simulink model "InterferenceModelingExample"  (Simulink 10.1)
settings: Solver=FixedStepDiscrete  StartTime=0.0  StopTime=1  RelTol=1e-3
undefined symbols (not defined in the file or in its folder): designMultirateFIR
libraries: commrflib2 x8, commdigbbndpm3 x2, commfilt2 x2, commrandsrc3 x2, commsink2 x1, commrfcorlib x1, commsync2 x1, commdigbbndcpm2 x1, dspsigattribs x1, dspmlti4 x1
settings Model: Creator=The MathWorks, Inc.  LastModifiedBy=iba
settings DataIOCC: SaveFormat=Dataset  ReturnWorkspaceOutputs=on
settings OptimizationCC: EfficientMapNaN2IntZero=off  LifeSpan=auto
settings DebuggingCC: UnderspecifiedInitializationDetection=Simplified  MergeDetectMultiDrivingBlocksExec=error  SFUnexpectedBacktrackingDiag=error  SFNoUnconditionalDefaultTransitionDiag=error  SFExecutionAtInitializationDiag=warning  ArithmeticOperatorsInVariantConditions=error
settings HardwareCC: ProdBitPerPointer=64  ProdBitPerSizeT=64  ProdBitPerPtrDiffT=64  ProdLargestAtomicFloat=Float  ProdIntDivRoundTo=Zero  ProdEndianess=LittleEndian  ProdWordSize=64  ProdHWDeviceType=Intel->x86-64 (Windows64)  TargetBitPerPointer=64  TargetBitPerSizeT=64  TargetBitPerPtrDiffT=64  TargetLongLongMode=on  TargetIntDivRoundTo=Zero  TargetEndianess=LittleEndian  TargetWordSize=64  TargetHWDeviceType=MATLAB Host  ProdEqTarget=off
settings ModelReferenceCC: PropagateSignalLabelsOutOfModel=on
settings SFSimCC: SimUseLocalCustomCode=on
settings RTWCC: RTWUseLocalCustomCode=on
settings CodeAppCC: MaxIdLength=128  StateflowObjectComments=off
settings ConfigComp: CovMetricSettings=dwe  CovHtmlReporting=off  CovSaveCumulativeToWorkspaceVar=off  CovSaveSingleToWorkspaceVar=off  CovExternalEMLEnable=on

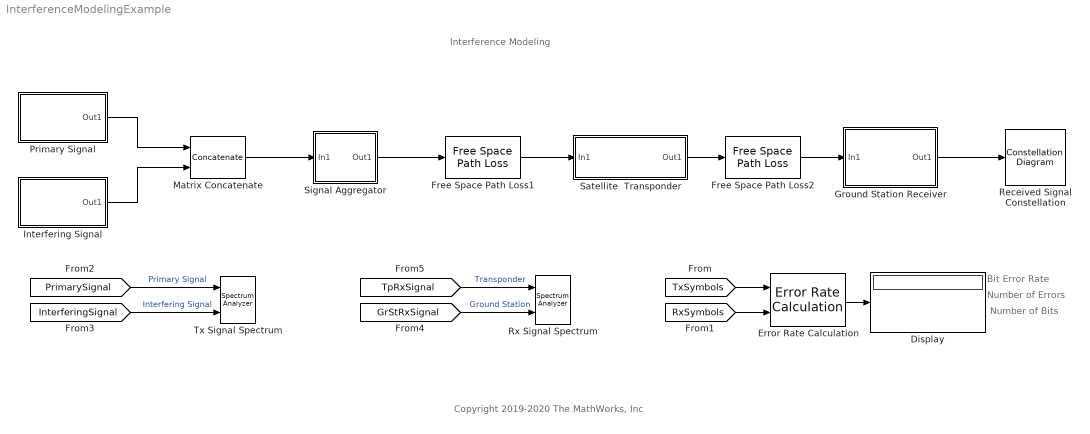
== system InterferenceModelingExample ==
  note: Interference Modeling
  note: Copyright 2019-2020 The MathWorks, Inc
  note: Bit Error Rate
  note: Number of Errors
  note: Number of Bits
  Display : Display
  Error Rate Calculation : commsink2/Error Rate Calculation  N=16 % 10  st_delay=0  cp_mode=Entire frame  subframe=[]  PMode=Port  WsName=ErrorVec  RsMode2=off  stop=off  numErr=100  maxBits=1e6
  Free Space Path Loss1 : commrflib2/Free Space Path Loss  mode=Decibels  dB=200  d=0.100  fc=1920
      settings: SourceProductBaseCode=CM
  Free Space Path Loss2 : commrflib2/Free Space Path Loss  mode=Decibels  dB=200  d=0.100  fc=1920
      settings: SourceProductBaseCode=CM
  Ground Station Receiver : Subsystem
      mask Display: disp('Ground Station\nReceiver')
  Interfering Signal : Subsystem
      mask Display: disp('Interfering\nSignal')
  Matrix Concatenate : Concatenate  Mode=Multidimensional array  ConcatenateDimension=2
  Primary Signal : Subsystem
      mask Display: disp('Primary\nSignal')
  Received Signal Constellation : ConstellationDiagram
  Rx Signal Spectrum : SpectrumAnalyzer  NumInputPorts=2
  Satellite  Transponder : Subsystem
      mask Display: disp('Satellite\nTransponder')
  Signal Aggregator : Subsystem  mask(Signal Aggregator){InterpolationMode=Auto, InputSampleRate=1e6, CenterFrequency=[0 400e3]}
      mask prompts: InterpolationMode "Interpolation mode:"; InputSampleRate "Sample rate of input signal (Hz):"; CenterFrequency "Desired output center frequencys (Hz):"
      mask help: Frequency shift input signals and aggregate them. Optionally, before frequency shifting the input signals, interpolate them such that the bandwidth of the aggregate output signal includes all the input signals.
      mask init:
      | Lnew = signalAggregator_MaskInit(gcbh, 'init', InterpolationMode, ...
      |     InputSampleRate, CenterFrequency);
      mask TypeOptions InterpolationMode: None | Auto
      mask Callback InterpolationMode: signalAggregator_MaskInit(gcbh, 'interpolationMode');
      mask Display: disp('Signal\nAggregator')
  Tx Signal Spectrum : SpectrumAnalyzer  NumInputPorts=2
  wires:
  Error Rate Calculation/1 -> Display/1
  Signal Aggregator/1(Out1) -> Free Space Path Loss1/1
  Free Space Path Loss1/1 -> Satellite  Transponder/1(In1)
  Satellite  Transponder/1(Out1) -> Free Space Path Loss2/1
  Ground Station Receiver/1(Out1) -> Received Signal Constellation/1
  [PrimarySignal] -> Tx Signal Spectrum/1  "Primary Signal"
  [InterferingSignal] -> Tx Signal Spectrum/2  "Interfering Signal"
  Primary Signal/1(Out1) -> Matrix Concatenate/1
  Interfering Signal/1(Out1) -> Matrix Concatenate/2
  Matrix Concatenate/1 -> Signal Aggregator/1(In1)
  [RxSymbols] -> Error Rate Calculation/2
  [TxSymbols] -> Error Rate Calculation/1
  [TpRxSignal] -> Rx Signal Spectrum/1  "Transponder"
  Free Space Path Loss2/1 -> Ground Station Receiver/1(In1)
  [GrStRxSignal] -> Rx Signal Spectrum/2  "Ground Station"

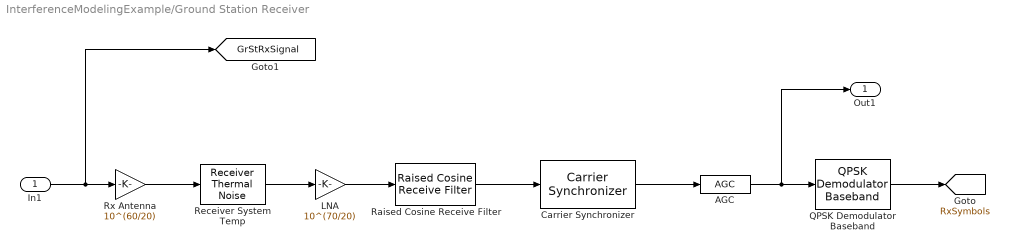
== system InterferenceModelingExample/Ground Station Receiver ==
  In1 : Inport
  AGC : commrfcorlib/AGC  LegacyMode=off  DetectorMethod=Rectifier  LoopMethod=Linear  UpdatePeriod=100  StepSize=0.1  AdaptationStepSize=0.01  DesiredOutputPower=1  AveragingLength=200  MaximumGain=30  MaxPowerGain=60  GainOutputPort=off  InputPowerOutputPort=off  SimulateUsing=Interpreted execution
  Carrier Synchronizer : commsync2/Carrier Synchronizer  Modulation=QPSK  ModulationPhaseOffset=Auto  CustomPhaseOffset=0  SamplesPerSymbol=1  DampingFactor=0.707  NormalizedLoopBandwidth=0.01  EstimatedPhaseErrorOutputPort=off  SimulateUsing=Code generation
  LNA : Gain  Gain=10^(70/20)
  QPSK Demodulator Baseband : commdigbbndpm3/QPSK Demodulator Baseband  OutType=Integer  DecType=Log-likelihood ratio  VarSource=Dialog  Variance=1  Dec=Gray  Ph=pi/4  outDtype1=Inherit via internal rule  outDtype2=Inherit via internal rule  derotateFactorWordLen=16  derotateFactorDataTypeStr=Inherit: Same word length as input  derotateFactorLastDataTypeStr=Inherit: Same word length as input
  Raised Cosine Receive Filter : commfilt2/Raised Cosine Receive Filter  filtType=Square root  R=.3  filtSpan=10  N=4  downFactor=4  downOffset=0  filterGain=1  InputProcessing=Columns as channels (frame based)  RateOptions=Enforce single-rate processing  framing=Mute  checkCoeff=off  variableName=rcRxFilt  currentFiltSpan=10  D=5  inputOffset=0  sampMode=Mute  saveAsFlag=0  rateMode=Downsampling  checkGain=Normalized  launchFVT=on  roundingMode=Floor  overflowMode=off  coeffDataTypeStr=Inherit: Same word length as input  coeffMin=[]  coeffMax=[]  coeffLastDataTypeStr=Inherit: Same word length as input  accumDataTypeStr=Inherit: Same as product output  accumLastDataTypeStr=Inherit: Same as product output  outputDataTypeStr=Inherit: Same as accumulator  outputMin=[]  outputMax=[]  outputLastDataTypeStr=Inherit: Same as accumulator
  Receiver System Temp : commrflib2/Receiver Thermal Noise  method=Noise temperature  ntemp=75  nfigure=20  nfactor=2  add290KAntennaNoise=off  seed=67987
      settings: SourceProductBaseCode=CM
  "Rx Antenna " : Gain  Gain=10^(60/20)  SaturateOnIntegerOverflow=on  OutDataTypeStr=Inherit: Same as input  ParamDataTypeStr=Inherit: Same as input
  Out1 : Outport  VectorParamsAs1DForOutWhenUnconnected=off
  tag scope: GrStRxSignal=global, RxSymbols=global
  wires:
  In1/1 -> [GrStRxSignal], "Rx Antenna "/1
  Raised Cosine Receive Filter/1 -> Carrier Synchronizer/1
  Receiver System Temp/1 -> LNA/1
  Carrier Synchronizer/1 -> AGC/1
  "Rx Antenna "/1 -> Receiver System Temp/1
  LNA/1 -> Raised Cosine Receive Filter/1
  AGC/1 -> QPSK Demodulator Baseband/1, Out1/1
  QPSK Demodulator Baseband/1 -> [RxSymbols]

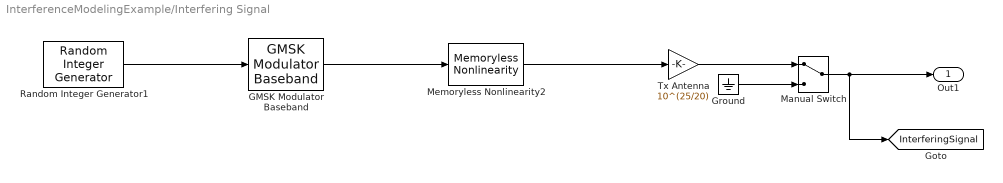
== system InterferenceModelingExample/Interfering Signal ==
  GMSK Modulator Baseband : commdigbbndcpm2/GMSK Modulator Baseband  inputType=Bit  BT=.3  pulseLength=4  preHistory=1  phaseOffset=0  samplesPerSymbol=8  RateOptions=Enforce single-rate processing  outDataType=double
      settings: SourceProductBaseCode=CM
  Ground : Ground
  Manual Switch : ManualSwitch
  Memoryless Nonlinearity2 : commrflib2/Memoryless Nonlinearity  model_select=Cubic polynomial  linGaindB=39  GindB=0  iip3=43  am2pm=.8  LPwrLimAMPM=-2.5  UPwrLimAMPM=17.5  amam=[2.1587 1.1517]  ampm=[4.0033 9.1040]  x=[8.1081 1.5413 6.5202 -0.0718]  y=[4.6645 2.0965 10.88 -0.003]  p=0.5  GoutdB=0  vsat=1
      settings: SourceProductBaseCode=CM
  Random Integer Generator1 : commrandsrc3/Random Integer Generator  SetSize=2  SeedSource=Auto  Seed=0  SampleTime=4/(500e3)  SamplesPerFrame=100  OutputDataType=boolean  SimulateUsing=Interpreted execution
  Tx Antenna : Gain  Gain=10^(25/20)  SaturateOnIntegerOverflow=on  OutDataTypeStr=Inherit: Same as input  ParamDataTypeStr=Inherit: Same as input
  Out1 : Outport  VectorParamsAs1DForOutWhenUnconnected=off
  tag scope: InterferingSignal=global
  wires:
  Memoryless Nonlinearity2/1 -> Tx Antenna/1
  Ground/1 -> Manual Switch/2
  Manual Switch/1 -> Out1/1, [InterferingSignal]
  Tx Antenna/1 -> Manual Switch/1
  GMSK Modulator Baseband/1 -> Memoryless Nonlinearity2/1
  Random Integer Generator1/1 -> GMSK Modulator Baseband/1

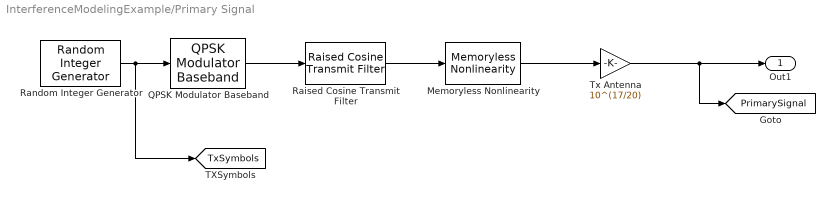
== system InterferenceModelingExample/Primary Signal ==
  Memoryless Nonlinearity : commrflib2/Memoryless Nonlinearity  model_select=Cubic polynomial  linGaindB=28  GindB=0  iip3=43  am2pm=.8  LPwrLimAMPM=-2.5  UPwrLimAMPM=17.5  amam=[2.1587 1.1517]  ampm=[4.0033 9.1040]  x=[8.1081 1.5413 6.5202 -0.0718]  y=[4.6645 2.0965 10.88 -0.003]  p=0.5  GoutdB=0  vsat=1
      settings: SourceProductBaseCode=CM
  QPSK Modulator Baseband : commdigbbndpm3/QPSK Modulator Baseband  InType=Integer  Enc=Gray  Ph=pi/4  outDtype=double  outWordLen=16  outUDDataType=sfix(16)  outFracLenMode=Best precision  outFracLen=15  outDataTypeStr=double  outLastDataTypeStr=double
  Raised Cosine Transmit Filter : commfilt2/Raised Cosine Transmit Filter  filtType=Square root  R=.3  filtSpan=10  N=2  filterGain=1  InputProcessing=Columns as channels (frame based)  RateOptions=Enforce single-rate processing  framing=Mute  checkCoeff=off  variableName=rcTxFilt  checkGain=Normalized  sampMode=Mute  saveAsFlag=0  currentFiltSpan=10  D=(10)/2  launchFVT=on  roundingMode=Floor  overflowMode=off  coeffDataTypeStr=Inherit: Same word length as input  coeffMin=[]  coeffMax=[]  coeffLastDataTypeStr=Inherit: Same word length as input  outputDataTypeStr=Inherit: Same as accumulator  outputMin=[]  outputMax=[]  outputLastDataTypeStr=Inherit: Same as accumulator
  Random Integer Generator : commrandsrc3/Random Integer Generator  SetSize=4  SeedSource=Auto  Seed=0  SampleTime=1/(500e3)  SamplesPerFrame=400  OutputDataType=double  SimulateUsing=Interpreted execution
  Tx Antenna : Gain  Gain=10^(17/20)  SaturateOnIntegerOverflow=on  OutDataTypeStr=Inherit: Same as input  ParamDataTypeStr=Inherit: Same as input
  Out1 : Outport  VectorParamsAs1DForOutWhenUnconnected=off
  tag scope: PrimarySignal=global, TxSymbols=global
  wires:
  QPSK Modulator Baseband/1 -> Raised Cosine Transmit Filter/1
  Random Integer Generator/1 -> [TxSymbols], QPSK Modulator Baseband/1
  Tx Antenna/1 -> [PrimarySignal], Out1/1
  Raised Cosine Transmit Filter/1 -> Memoryless Nonlinearity/1
  Memoryless Nonlinearity/1 -> Tx Antenna/1

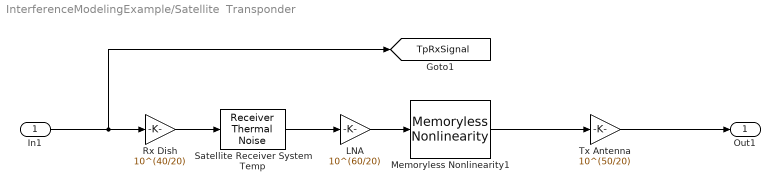
== system InterferenceModelingExample/Satellite  Transponder ==
  In1 : Inport
  LNA : Gain  Gain=10^(60/20)
  Memoryless Nonlinearity1 : commrflib2/Memoryless Nonlinearity  model_select=Cubic polynomial  linGaindB=66  GindB=0  iip3=51  am2pm=.8  LPwrLimAMPM=-7.5  UPwrLimAMPM=12.5  amam=[2.1587 1.1517]  ampm=[4.0033 9.1040]  x=[8.1081 1.5413 6.5202 -0.0718]  y=[4.6645 2.0965 10.88 -0.003]  p=0.5  GoutdB=0  vsat=1
      settings: SourceProductBaseCode=CM
  Rx Dish : Gain  Gain=10^(40/20)  SaturateOnIntegerOverflow=on  OutDataTypeStr=Inherit: Same as input  ParamDataTypeStr=Inherit: Same as input
  Satellite Receiver System Temp : commrflib2/Receiver Thermal Noise  method=Noise temperature  ntemp=30  nfigure=20  nfactor=2  add290KAntennaNoise=off  seed=67987
      settings: SourceProductBaseCode=CM
  Tx Antenna : Gain  Gain=10^(50/20)  SaturateOnIntegerOverflow=on  OutDataTypeStr=Inherit: Same as input  ParamDataTypeStr=Inherit: Same as input
  Out1 : Outport  VectorParamsAs1DForOutWhenUnconnected=off
  tag scope: TpRxSignal=global
  wires:
  LNA/1 -> Memoryless Nonlinearity1/1
  Memoryless Nonlinearity1/1 -> Tx Antenna/1
  Tx Antenna/1 -> Out1/1
  In1/1 -> [TpRxSignal], Rx Dish/1
  Rx Dish/1 -> Satellite Receiver System Temp/1
  Satellite Receiver System Temp/1 -> LNA/1

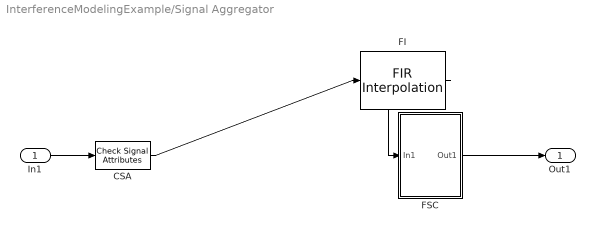
== system InterferenceModelingExample/Signal Aggregator ==
  In1 : Inport
  CSA : dspsigattribs/Check Signal Attributes  SigAttribCheckMethod=Does not match attributes exactly  Complexity=Ignore  Frame=Ignore  DimsCheckMethod=Ignore  Dimensions=Full matrix (2-D)  DatatypeCheckMethod=Ignore  DatatypeGeneral=Boolean  DtypeFloatSpecific=Any floating-point  DtypeFixedSpecific=Any fixed-point  DtypeIntSpecific=Any integer  SampleMode=Discrete
      settings: SourceProductBaseCode=DS
  FI : dspmlti4/FIR Interpolation  FilterSource=Auto  PrivateCoeffs=0  h=designMultirateFIR(3,1)  L=Lnew  FilterObject=FINTERP  InputProcessing=Columns as channels (frame based)  framing=Enforce single-rate processing  outputBufInitCond=0  roundingMode=Floor  overflowMode=off  firstCoeffDataTypeStr=Inherit: Same word length as input  firstCoeffMin=[]  firstCoeffMax=[]  firstCoeffLastDataTypeStr=Inherit: Same word length as input  outputDataTypeStr=Inherit: Same as accumulator  outputMin=[]  outputMax=[]  outputLastDataTypeStr=Inherit: Same as accumulator
  FSC : Subsystem  mask{CenterFrequency=CenterFrequency}
      mask prompts: CenterFrequency "Desired output center frequency (Hz):"
      mask help: Shift the frequency of input matrix signal and combine all the signals in the input matrix into one signal.
  Out1 : Outport
  wires:
  FSC/1(Out1) -> Out1/1
  In1/1 -> CSA/1
  CSA/1 -> FI/1
  FI/1 -> FSC/1(In1)

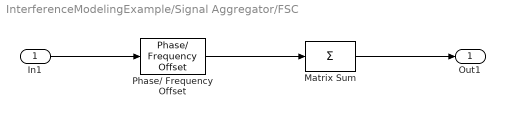
== system InterferenceModelingExample/Signal Aggregator/FSC ==
  In1 : Inport
  Matrix Sum : Sum  Inputs=+  CollapseMode=Specified dimension  CollapseDim=2
  Phase/ Frequency Offset : commrflib2/Phase// Frequency Offset  phaseOffset=0  freqPort=off  freqOffset=CenterFrequency
  Out1 : Outport
  wires:
  Matrix Sum/1 -> Out1/1
  In1/1 -> Phase/ Frequency Offset/1
  Phase/ Frequency Offset/1 -> Matrix Sum/1
